simulink model "pendbasic"  (Simulink 7.1)
settings: Solver=ode5  StartTime=0.0  StopTime=10  FixedStep=h  RelTol=1e-3
values from neighbouring files (symbols this model uses):
  Fscomp_neg = 0.16    [pendinit.m]
  Fscomp_pos = 0.16    [pendinit.m]
  g = 9.81    [pendinit.m]
  h = 0.01    [pendinit.m]
  J = 0.05    [pendinit.m]
  Jp = 0.0009    [pendinit.m]
  l = 0.413    [pendinit.m]
  Lnopos = dlqr(Afd,Bfd,Q,R)    [pendinit.m]
  Lpos = dlqr(Afd,Bfd,Q,R)    [pendinit.m]
  M = 0.01    [pendinit.m]
  m = 0.02    [pendinit.m]
  r = 0.235    [pendinit.m]
  x0 = x_0    [furuta.m]    (also in pendinit.m = [0.1 0 0 0]')
libraries: simulink3 x2
settings Model: Creator=lincoln  LastModifiedBy=martink  ExtModeTrigMode=oneshot  ExtModeArmWhenConnect=off  ExtModeAutoUpdateStatusClock=off
settings DataIOCC: LimitDataPoints=off
settings OptimizationCC: BooleanDataType=off
settings DebuggingCC: SaveWithParameterizedLinksMsg=none  SignalResolutionControl=TryResolveAllWithWarning  SolverPrmCheckMsg=none  MultiTaskDSMMsg=warning  MultiTaskCondExecSysMsg=none  StrictBusMsg=None
settings HardwareCC: TargetUnknown=on
settings RTWCC: IncludeERTFirstTime=on

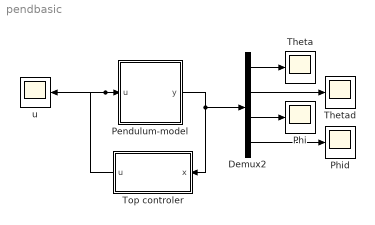
== system pendbasic ==
  Demux2 : Demux
  Pendulum-model : Subsystem
      mask Display: disp('Model')
  Phi : Scope
      settings: TimeRange=25  YMin=-0.0004  YMax=5e-05
  Phid : Scope
  Theta : Scope
      settings: YMin=-0.02  YMax=0.02
  Thetad : Scope
  Top controler : Subsystem  Orientation=left
  u : Scope
      settings: YMin=-1  YMax=1.25
  wires:
  Top controler/1(u) -> u/1, Pendulum-model/1(u)
  Demux2/2 -> Thetad/1
  Demux2/3 -> Phi/1
  Demux2/4 -> Phid/1
  Demux2/1 -> Theta/1
  Pendulum-model/1(y) -> Demux2/1, Top controler/1(x)

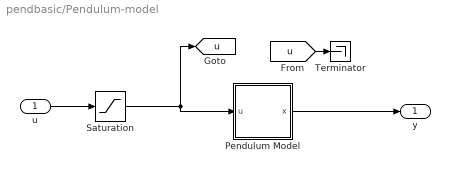
== system pendbasic/Pendulum-model ==
  u : Inport
  Pendulum Model : Subsystem
  Saturation : Saturate  UpperLimit=2  LowerLimit=-2
  Terminator : Terminator
  y : Outport  InitialOutput=0
  tag scope: u=global
  wires:
  Pendulum Model/1(x) -> y/1
  [u] -> Terminator/1
  u/1 -> Saturation/1
  Saturation/1 -> [u], Pendulum Model/1(u)

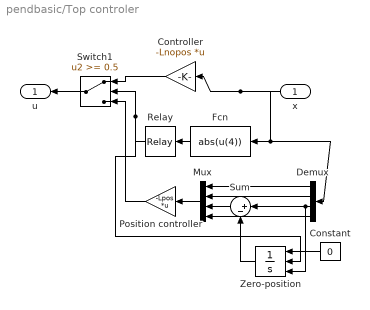
== system pendbasic/Top controler ==
  x : Inport  Orientation=left
  Constant : Constant  Orientation=left  Value=0
  Controller : Gain  Orientation=left  Gain=-Lnopos  Multiplication=Matrix(K*u)  SaturateOnIntegerOverflow=on  OutDataTypeStr=Inherit: Same as input  ParamDataTypeStr=Inherit: Same as input
  Demux : Demux  Orientation=left
  Fcn : Fcn  Orientation=left  Expr=abs(u(4))
  Mux : Mux  Orientation=left
  Position controller : Gain  Orientation=left  Gain=-Lpos  Multiplication=Matrix(K*u)  SaturateOnIntegerOverflow=on  OutDataTypeStr=Inherit: Same as input  ParamDataTypeStr=Inherit: Same as input
  Relay : Relay  Orientation=left  OnSwitchValue=4  OffSwitchValue=3.9
  Sum : Sum  Orientation=left  Inputs=|+-  SaturateOnIntegerOverflow=on  InputSameDT=on  OutDataTypeStr=Inherit: Same as first input
  Switch1 : Switch  Orientation=left  Threshold=0.5  SaturateOnIntegerOverflow=on  InputSameDT=on
  Zero-position : Integrator  Orientation=left  ExternalReset=falling  InitialConditionSource=external
  u : Outport  Orientation=left
  wires:
  Switch1/1 -> u/1
  Sum/1 -> Mux/3
  Zero-position/1 -> Sum/2
  Fcn/1 -> Relay/1
  Constant/1 -> Zero-position/1
  Demux/3 -> Sum/1, Zero-position/3
  Demux/4 -> Mux/4
  Demux/2 -> Mux/2
  Demux/1 -> Mux/1
  Mux/1 -> Position controller/1
  Controller/1 -> Switch1/1
  Relay/1 -> Zero-position/2, Switch1/2
  Position controller/1 -> Switch1/3
  x/1 -> Demux/1, Fcn/1, Controller/1

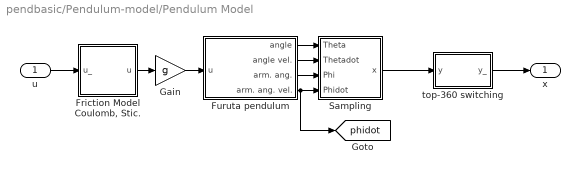
== system pendbasic/Pendulum-model/Pendulum Model ==
  u : Inport
  "Friction Model Coulomb, Stic." : Subsystem
  Furuta pendulum : Subsystem  mask{l=l, M=M, Jp=Jp, r=r, J=J, m_w=m, g=g, x_0=x0}
      mask prompts: l "Pendulum Length"; M "Mass of Pendulum"; r "Length of Arm"; m_w "Mass of weight"
  Gain : Gain  Gain=g  SaturateOnIntegerOverflow=on  OutDataTypeStr=Inherit: Same as input  ParamDataTypeStr=Inherit: Same as input
  Sampling : Subsystem
  top-360 switching : Subsystem
  x : Outport  InitialOutput=0
  tag scope: phidot=global
  wires:
  top-360 switching/1(y_) -> x/1
  Sampling/1(x) -> top-360 switching/1(y)
  Furuta pendulum/1(angle) -> Sampling/1(Theta)
  Furuta pendulum/3(arm. ang.) -> Sampling/3(Phi)
  Furuta pendulum/2(angle vel.) -> Sampling/2(Thetadot)
  Furuta pendulum/4(arm. ang. vel.) -> Sampling/4(Phidot), [phidot]
  u/1 -> "Friction Model Coulomb, Stic."/1(u_)
  "Friction Model Coulomb, Stic."/1(u) -> Gain/1
  Gain/1 -> Furuta pendulum/1(u)

== system pendbasic/Pendulum-model/Pendulum Model/Friction Model Coulomb, Stic. ==
  u_ : Inport
  Friction model : Subsystem
  u : Outport  InitialOutput=0
  wires:
  Friction model/1(u_) -> u/1
  [phidot] -> Friction model/2(phidot)
  u_/1 -> Friction model/1(u)

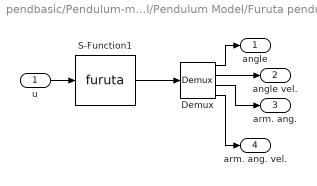
== system pendbasic/Pendulum-model/Pendulum Model/Furuta pendulum ==
  u : Inport
  Demux : Demux
  S-Function1 : S-Function  FunctionName=furuta  Parameters=l, M, Jp, r, J, m_w, g, x_0  EnableBusSupport=off
  angle : Outport  InitialOutput=0
  angle vel. : Outport  Port=2  InitialOutput=0
  arm. ang. : Outport  Port=3  InitialOutput=0
  arm. ang. vel. : Outport  Port=4  InitialOutput=0
  wires:
  Demux/4 -> arm. ang. vel./1
  Demux/3 -> arm. ang./1
  u/1 -> S-Function1/1
  Demux/2 -> angle vel./1
  Demux/1 -> angle/1
  S-Function1/1 -> Demux/1

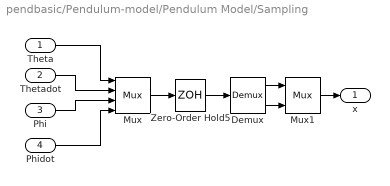
== system pendbasic/Pendulum-model/Pendulum Model/Sampling ==
  Theta : Inport
  Thetadot : Inport  Port=2
  Phi : Inport  Port=3
  Phidot : Inport  Port=4
  Demux : Demux  Outputs=[3 1]
  Mux : Mux
  Mux1 : Mux  Inputs=2
  Zero-Order Hold5 : ZeroOrderHold  SampleTime=h
  x : Outport  InitialOutput=0
  wires:
  Demux/2 -> Mux1/2
  Theta/1 -> Mux/1
  Thetadot/1 -> Mux/2
  Phi/1 -> Mux/3
  Phidot/1 -> Mux/4
  Mux/1 -> Zero-Order Hold5/1
  Zero-Order Hold5/1 -> Demux/1
  Mux1/1 -> x/1
  Demux/1 -> Mux1/1

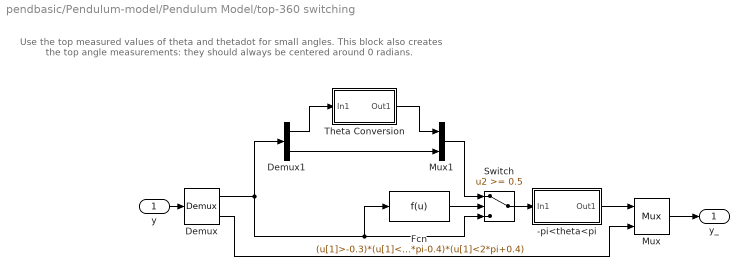
== system pendbasic/Pendulum-model/Pendulum Model/top-360 switching ==
  note: Use the top measured values of
      | theta and thetadot for small angles.
      | This block also creates the top angle
      | measurements: they should always be
      | centered around 0 radians.
  y : Inport
  -pi<theta<pi : Subsystem
  Demux : Demux  Outputs=[2 2]
  Demux1 : Demux  Outputs=2
  Fcn : Fcn  Expr=(u[1]>-0.3)*(u[1]<0.4)+(u[1]>2*pi-0.4)*(u[1]<2*pi+0.4)
  Mux : Mux  Inputs=2
  Mux1 : Mux  Inputs=2
  Switch : Switch  Threshold=0.5  SaturateOnIntegerOverflow=on  InputSameDT=on
  Theta Conversion : Subsystem
  y_ : Outport
  wires:
  Mux1/1 -> Switch/1
  Demux1/2 -> Mux1/2
  Demux1/1 -> Theta Conversion/1(In1)
  Demux/1 -> Fcn/1, Switch/3, Demux1/1
  Demux/2 -> Mux/2
  y/1 -> Demux/1
  Mux/1 -> y_/1
  Fcn/1 -> Switch/2
  Theta Conversion/1(Out1) -> Mux1/1
  Switch/1 -> -pi<theta<pi/1(In1)
  -pi<theta<pi/1(Out1) -> Mux/1

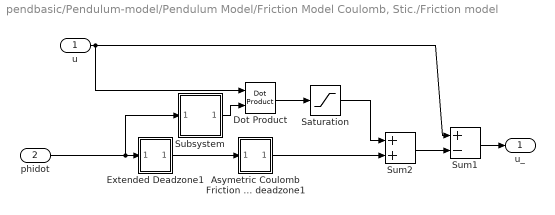
== system pendbasic/Pendulum-model/Pendulum Model/Friction Model Coulomb, Stic./Friction model ==
  u : Inport
  phidot : Inport  Port=2
  Asymetric Coulomb Friction with deadzone1 : Subsystem  mask{Fc_neg=Fscomp_neg, Fc_pos=Fscomp_pos, dv=0.04}
      mask prompts: Fc_neg "Coulomb Friction (Negative)"; Fc_pos "Coulomb Friction (Positive)"; dv "Deadzone width (Onesided)"
      mask Display:
      | plot([-1 0 0], [0 0 1], [0 0 1],[-1 0 0]);
      | plot([0.5 0.5 1],[0 0.5 0.5],[-0.5 -0.5 -1],[0 -0.5 -0.5]);
  Dot Product : simulink3/Math/Dot Product
  Extended Deadzone1 : Subsystem  mask{vg=1, dv=0.04}
      mask prompts: vg "Gain"; dv "Deadzone width (Onesided)"
      mask init:
      | v_gain=vg;
      | d_v=dv;
      mask Display:
      | plot([-1 0 0], [0 0 1], [0 0 1],[-1 0 0]);
      | plot([0.5 0.5 1],[0 0.5 1],[-0.5 -0.5 -1],[0 -0.5 -1]);
  Saturation : Saturate  UpperLimit=Fscomp_pos  LowerLimit=-Fscomp_neg
  Subsystem : Subsystem  mask{dw=0.04}
      mask prompts: dw "Width (Onesided)"
      mask init:
      | d_w=dw;
      mask Display:
      | plot([-1 0 0], [0 0 1], [0 0 1],[-0.3 0 0]);
      | plot([-0.5 -0.5 0.5 0.5],[0 0.7 0.7 0])
  Sum1 : Sum  Inputs=+-  SaturateOnIntegerOverflow=on  InputSameDT=on  OutDataTypeStr=Inherit: Same as first input
  Sum2 : Sum  SaturateOnIntegerOverflow=on  InputSameDT=on  OutDataTypeStr=Inherit: Same as first input
  u_ : Outport  InitialOutput=0
  wires:
  Asymetric Coulomb Friction with deadzone1/1(Out1) -> Sum2/2
  Sum2/1 -> Sum1/2
  u/1 -> Sum1/1, Dot Product/1
  Dot Product/1 -> Saturation/1
  Subsystem/1(Out1) -> Dot Product/2
  Extended Deadzone1/1(Out1) -> Asymetric Coulomb Friction with deadzone1/1(In1)
  Sum1/1 -> u_/1
  phidot/1 -> Subsystem/1(In1), Extended Deadzone1/1(In1)
  Saturation/1 -> Sum2/1

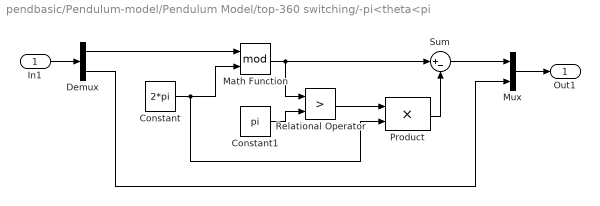
== system pendbasic/Pendulum-model/Pendulum Model/top-360 switching/-pi<theta<pi ==
  In1 : Inport
  Constant : Constant  Value=2*pi
  Constant1 : Constant  Value=pi
  Demux : Demux  Outputs=2
  Math Function : Math  Operator=mod  SaturateOnIntegerOverflow=on
  Mux : Mux  Inputs=2
  Product : Product  SaturateOnIntegerOverflow=on  RndMeth=Zero  InputSameDT=on  OutDataTypeStr=Inherit: Same as first input
  Relational Operator : RelationalOperator  Operator=>  InputSameDT=on
  Sum : Sum  Inputs=|+-  SaturateOnIntegerOverflow=on  InputSameDT=on  OutDataTypeStr=Inherit: Same as first input
  Out1 : Outport
  wires:
  Constant/1 -> Math Function/2, Product/2
  Math Function/1 -> Sum/1, Relational Operator/1
  Constant1/1 -> Relational Operator/2
  Relational Operator/1 -> Product/1
  Product/1 -> Sum/2
  In1/1 -> Demux/1
  Demux/1 -> Math Function/1
  Sum/1 -> Mux/1
  Mux/1 -> Out1/1
  Demux/2 -> Mux/2

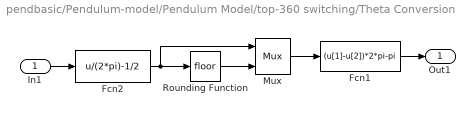
== system pendbasic/Pendulum-model/Pendulum Model/top-360 switching/Theta Conversion ==
  In1 : Inport
  Fcn1 : Fcn  Expr=(u[1]-u[2])*2*pi-pi
  Fcn2 : Fcn  Expr=u/(2*pi)-1/2
  Mux : Mux  Inputs=2
  Rounding Function : Rounding
  Out1 : Outport  InitialOutput=0
  wires:
  Rounding Function/1 -> Mux/2
  Fcn2/1 -> Rounding Function/1, Mux/1
  Mux/1 -> Fcn1/1
  Fcn1/1 -> Out1/1
  In1/1 -> Fcn2/1

== system pendbasic/Pendulum-model/Pendulum Model/Friction Model Coulomb, Stic./Friction model/Asymetric Coulomb Friction with deadzone1 ==
  In1 : Inport  Orientation=left
  Dead Zone : DeadZone  Orientation=left  LowerValue=-dv  UpperValue=dv  SaturateOnIntegerOverflow=on
  Fcn : Fcn  Orientation=left  Expr=(u<0)*u*Fc_neg+(u>0)*u*Fc_pos
  Sign : Signum  Orientation=left
  Out1 : Outport  Orientation=left  InitialOutput=0
  wires:
  In1/1 -> Dead Zone/1
  Dead Zone/1 -> Sign/1
  Sign/1 -> Fcn/1
  Fcn/1 -> Out1/1

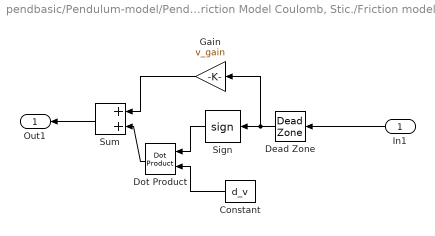
== system pendbasic/Pendulum-model/Pendulum Model/Friction Model Coulomb, Stic./Friction model/Extended Deadzone1 ==
  In1 : Inport  Orientation=left
  Constant : Constant  Orientation=left  Value=d_v
  Dead Zone : DeadZone  Orientation=left  LowerValue=-d_v  UpperValue=d_v  SaturateOnIntegerOverflow=on
  Dot Product : simulink3/Math/Dot Product  Orientation=left
  Gain : Gain  Orientation=left  Gain=v_gain  SaturateOnIntegerOverflow=on  OutDataTypeStr=Inherit: Same as input  ParamDataTypeStr=Inherit: Same as input
  Sign : Signum  Orientation=left
  Sum : Sum  Orientation=left  SaturateOnIntegerOverflow=on  InputSameDT=on  OutDataTypeStr=Inherit: Same as first input
  Out1 : Outport  Orientation=left  InitialOutput=0
  wires:
  Sum/1 -> Out1/1
  Dot Product/1 -> Sum/2
  Constant/1 -> Dot Product/2
  Dead Zone/1 -> Sign/1, Gain/1
  Sign/1 -> Dot Product/1
  In1/1 -> Dead Zone/1
  Gain/1 -> Sum/1

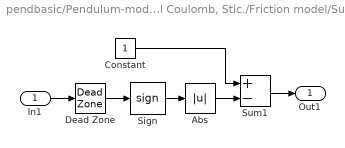
== system pendbasic/Pendulum-model/Pendulum Model/Friction Model Coulomb, Stic./Friction model/Subsystem ==
  In1 : Inport
  Abs : Abs  SaturateOnIntegerOverflow=on
  Constant : Constant
  Dead Zone : DeadZone  LowerValue=-d_w  UpperValue=d_w  SaturateOnIntegerOverflow=on
  Sign : Signum
  Sum1 : Sum  Inputs=+-  SaturateOnIntegerOverflow=on  InputSameDT=on  OutDataTypeStr=Inherit: Same as first input
  Out1 : Outport  InitialOutput=0
  wires:
  Abs/1 -> Sum1/2
  Sign/1 -> Abs/1
  Sum1/1 -> Out1/1
  Constant/1 -> Sum1/1
  In1/1 -> Dead Zone/1
  Dead Zone/1 -> Sign/1
